simulink model "TV_2017_HIL"  (R2016a)
settings: Solver=ode1  StartTime=0.0  StopTime=600  FixedStep=0.001  RelTol=1e-3
PreLoadFcn:
  | HIL_parameters
values from neighbouring files (symbols this model uses):
  battery_voltage = single(530)    [HIL_parameters.m]    (also in HIL_parameters_2018.m; TV_2017_parameters.m; TV_2017_parameters_VD.m)
  car_params = Simulink_Car_params    [HIL_parameters.m]    (also in HIL_parameters_2018.m; TV_2017_parameters.m; TV_2017_parameters_VD.m)
  i_Diff = 16    [HIL_parameters.m]    (also in HIL_parameters_2018.m; TV_2017_parameters.m)
  Kp = 1    [HIL_parameters.m]    (also in HIL_parameters_2018.m; TV_2017_parameters.m; TV_2017_parameters_VD.m)
  motor_data = struct    [HIL_parameters.m]    (also in HIL_parameters_2018.m; TV_2017_parameters.m)
  settings = Simulink_Settings    [HIL_parameters.m]    (also in HIL_parameters_2018.m; TV_2017_parameters.m; TV_2017_parameters_VD.m)
  SpdC_BCC = 0    [HIL_parameters.m]    (also in HIL_parameters_2018.m; TV_2017_parameters.m; TV_2017_parameters_VD.m)
  Speed_Neg_sat = -21    [HIL_parameters.m]    (also in HIL_parameters_2018.m; TV_2017_parameters.m; TV_2017_parameters_VD.m)
  Speed_Pos_sat = 21    [HIL_parameters.m]    (also in HIL_parameters_2018.m; TV_2017_parameters.m; TV_2017_parameters_VD.m)
  SteeringAngleFL = [-23.80 -22.65 -21.50 -20.34 -19.18 -18.03 -16.86 -15.70 -14.53 -13.35 -12.18 -10.99 -9.80 -8.61 -7.40 -6.19 -4.97 -3.75 -2.51 -1.26 0 1.27 2.56 3.85 5.17 6.50 7.84 9.21 10.59 12.00 13.42 14.88 16.36 17.87 19.41 20.99 22.61 24.26 25.97 27.73 29.54]    [CarSetupAnalysis2018.m]    (also in HIL_parameters_2018.m; TV_2017_parameters.m; TV_2017_parameters_VD.m = [-24.129 -22.950 -21.772 -20.593 -19.413 -18.232 -17.050 -15)
  SteeringAngleFR = [-29.54 -27.73 -25.97 -24.26 -22.61 -20.99 -19.41 -17.87 -16.36 -14.88 -13.42 -12.00 -10.59 -9.21 -7.84 -6.50 -5.17 -3.85 -2.56 -1.27 0 1.26 2.51 3.75 4.97 6.19 7.40 8.61 9.80 10.99 12.18 13.35 14.53 15.70 16.86 18.03 19.18 20.34 21.50 22.65 23.80]    [CarSetupAnalysis2018.m]    (also in HIL_parameters_2018.m; TV_2017_parameters.m; TV_2017_parameters_VD.m = [-29.3050 -27.5340 -25.8140 -24.1410 -22.5110 -20.9180 -19.3)
  SteeringWhAngle = [-105 -99.75 -94.5 -89.25 -84 -78.75 -73.5 -68.25 -63 -57.75 -52.5 -47.25 -42 -36.75 -31.5 -26.25 -21.0 -15.75 -10.5 -5.25 0.0 5.25 10.50 15.75 21.00 26.25 31.50 36.75 42.00 47.25 52.50 57.75  63.00 68.25 73.50 78.75 84.00 89.25 94.50 99.75 105.00]    [TV_2017_parameters_VD.m]
  Tn_n = 0    [HIL_parameters.m]    (also in HIL_parameters_2018.m; TV_2017_parameters.m; TV_2017_parameters_VD.m)
  Use_Joystick = 1    [HIL_parameters.m]    (also in HIL_parameters_2018.m; TV_2017_parameters.m; TV_2017_parameters_VD.m)
undefined symbols (not defined in the file or in its folder): canChannel, TC_Decr_Gas, TC_Derivative, TC_Incr_Gas, TC_On, TC_Relay_Off, TC_Relay_On
libraries: CarMaker4SL x314, canmsglib x48, simulink_extras x48, simulink x41, canlib x39, powerlib_meascontrol x2, sldrtlib x1
(part 2 of 9)

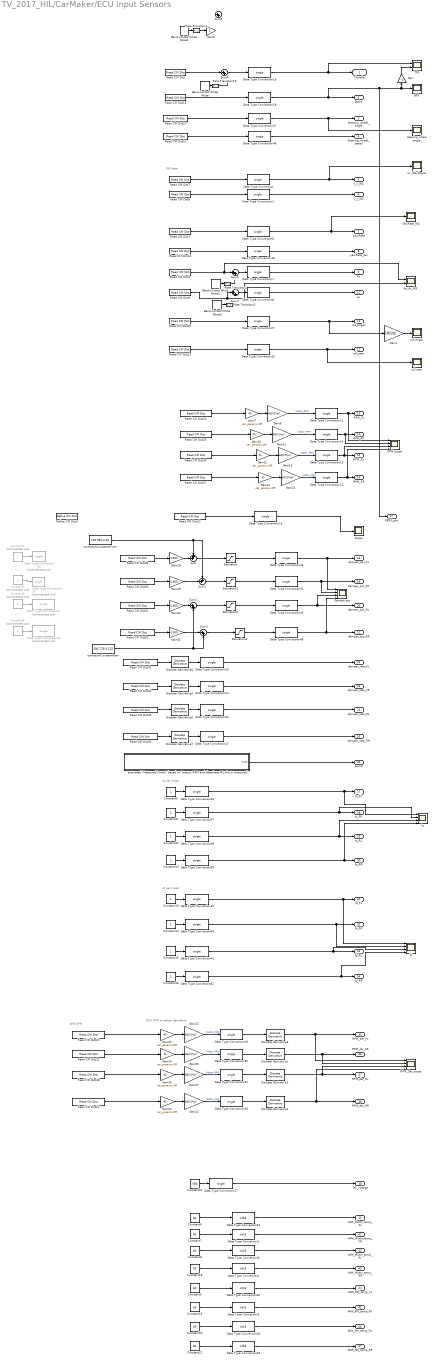
== system TV_2017_HIL/CarMaker/ECU input Sensors  ==
  note: INS data
  note: ECU RPM to radian derivative
  note: AMK RPM
  note: Id per motor
  note: Iq per motor
  Ay_Ax_INS : Scope  NumInputPorts=2
  BPS : Scope
  Band-Limited White Noise : simulink/Sources/Band-Limited White Noise  Cov=[0.00002]  Ts=0.1  seed=[23341]
  Band-Limited White Noise1 : simulink/Sources/Band-Limited White Noise  Cov=[0.00002]  Ts=0.1  seed=[23341]
  Band-Limited White Noise2 : simulink/Sources/Band-Limited White Noise  Cov=[0.01]  Ts=0.1  seed=[23341]
  Band-Limited White Noise3 : simulink/Sources/Band-Limited White Noise  Cov=[0.01]  Ts=0.1  seed=[23341]
  Constant{1..4} (4 alike) : Constant  Commented=on
  Constant{9..16} (8 alike) : Constant
  Constant{5..8,18..20,22} (8 alike) : Constant  Value=60
  Constant21 : Constant  Value=580
  Damper pos : Scope  NumInputPorts=4
  Data Type Conversion{,1,6..19,24..27,32..33,37..52} (38 alike) : DataTypeConversion  OutDataTypeStr=single
  Data Type Conversion{2..5,28..30,54} (8 alike) : DataTypeConversion  OutDataTypeStr=int16
  Data Type Conversion{20..23} (4 alike) : DataTypeConversion  Commented=on  OutDataTypeStr=single
  Define CM Dict3 : CarMaker4SL/Define CM Dict  xname=KERS_pos  xmono=off  xtype=Double  xdvaplace=None  xnstates=0  xfirststate=0  xinitial=0
  Discrete Derivative{1..3,8} (4 alike) : simulink/Discrete/Discrete Derivative  gainval=1.0  ICPrevScaledInput=0.0  InputProcessing=Inherited  OutMin=[]  OutMax=[]  OutDataType=fixdt(1, 16)  OutScaling=2^-10  DoSatur=off
  Discrete Derivative{4..7} (4 alike) : simulink/Discrete/Discrete Derivative  gainval=1.0  ICPrevScaledInput=0.0  OutMin=[]  OutMax=[]  OutDataType=fixdt(1, 16)  OutScaling=2^-10  DoSatur=off
  Gain : Gain  Gain=-1
  Gain1 : Gain  Gain=180/pi
  Gain{7,10,12,14,20,22,24,26} (8 alike) : Gain  Gain=car_params.GR
  Gain{9,11,13,15,21,23,25,27} (8 alike) : Gain  Gain=60/(2*pi)
  Gain2 : Gain
  Gain{28..31} (4 alike) : Gain  Gain=-1000
  Id : Scope  NumInputPorts=4
  Iq : Scope  NumInputPorts=4
  RPM scope : Scope  NumInputPorts=4
  "RPM_Der_scope " : Scope  NumInputPorts=4
  Rate Transition{1..3,19} (4 alike) : RateTransition  OutPortSampleTimeOpt=Inherit  OutPortSampleTime=matlab_params.sensor_sampling_time
  Read CM Dict : CarMaker4SL/Read CM Dict  xname=VC.Gas  xsync=off
  Read CM Dict1 : CarMaker4SL/Read CM Dict  xname=Vhcl.YawRate  xsync=off
  Read CM Dict10 : CarMaker4SL/Read CM Dict  xname=Vhcl.Roll  xsync=off
  Read CM Dict11 : CarMaker4SL/Read CM Dict  xname=Vhcl.RollVel  xsync=off
  Read CM Dict12 : CarMaker4SL/Read CM Dict  xname=KERS_pos  xsync=off
  Read CM Dict13 : CarMaker4SL/Read CM Dict  xname=Vhcl.YawAcc  xsync=off
  Read CM Dict14 : CarMaker4SL/Read CM Dict  xname=Car.WheelSpd_RR  xsync=off
  Read CM Dict15 : CarMaker4SL/Read CM Dict  xname=VC.Brake  xsync=off
  Read CM Dict2 : CarMaker4SL/Read CM Dict  xname=Car.ay  xsync=off
  Read CM Dict20 : CarMaker4SL/Read CM Dict  xname=Vhcl.Steer.Ang  xsync=off
  Read CM Dict21 : CarMaker4SL/Read CM Dict  xname=Vhcl.Steer.Vel  xsync=off
  Read CM Dict22 : CarMaker4SL/Read CM Dict  xname=Car.WheelSpd_FL  xsync=off
  Read CM Dict23 : CarMaker4SL/Read CM Dict  xname=Car.WheelSpd_FR  xsync=off
  Read CM Dict24 : CarMaker4SL/Read CM Dict  xname=Car.WheelSpd_FL  xsync=off
  Read CM Dict25 : CarMaker4SL/Read CM Dict  xname=Car.WheelSpd_FR  xsync=off
  Read CM Dict26 : CarMaker4SL/Read CM Dict  xname=Car.WheelSpd_RL  xsync=off
  Read CM Dict27 : CarMaker4SL/Read CM Dict  xname=Car.WheelSpd_RR  xsync=off
  Read CM Dict28 : CarMaker4SL/Read CM Dict  xname=Car.WheelSpd_RL  xsync=off
  Read CM Dict29 : CarMaker4SL/Read CM Dict  xname=Car.SpringFL.l  xsync=off
  Read CM Dict30 : CarMaker4SL/Read CM Dict  xname=Car.SpringFR.l  xsync=off
  Read CM Dict31 : CarMaker4SL/Read CM Dict  xname=Car.SpringRL.l  xsync=off
  Read CM Dict32 : CarMaker4SL/Read CM Dict  xname=Car.SpringRR.l  xsync=off
  Read CM Dict33 : CarMaker4SL/Read CM Dict  xname=Car.SpringFL.l  xsync=off
  Read CM Dict34 : CarMaker4SL/Read CM Dict  xname=Car.SpringFR.l  xsync=off
  Read CM Dict35 : CarMaker4SL/Read CM Dict  xname=Car.SpringRL.l  xsync=off
  Read CM Dict36 : CarMaker4SL/Read CM Dict  xname=Car.SpringRR.l  xsync=off
  Read CM Dict7 : CarMaker4SL/Read CM Dict  xname=Car.vx  xsync=off
  Read CM Dict8 : CarMaker4SL/Read CM Dict  xname=Car.vy  xsync=off
  Read CM Dict9 : CarMaker4SL/Read CM Dict  xname=Car.ax  xsync=off
  Saturation{,1..3} (4 alike) : Saturate  UpperLimit=200  LowerLimit=0.001
  Scope : Scope
  Sum : Sum  Inputs=++|
  Sum1 : Sum  Inputs=++|
  Sum{2..7} (6 alike) : Sum  Inputs=|++
  TPS : Scope  NumInputPorts=2
  Vx_INS_Scope : Scope
  YawRate_INS : Scope
  correctionConstantRear : Constant  Value=190.725-3.125
  correctionCornstantFront : Constant  Value=190.965-3.63
  "estimated \"Measured Power\" based on Torque, RPM and datasheet IRL this is measured" : Subsystem
  "roll angle " : Scope
  roll rate : Scope
  steering wheel angle : Scope
  "Throttle " : Outport
  "Brake " : Outport  Port=2
  "Steering_wheel_angle " : Outport  Port=3
  Steering_wheel_speed : Outport  Port=4
  V_x_INS : Outport  Port=5
  V_y_INS : Outport  Port=6
  yawRate : Outport  Port=7
  yawRate_der : Outport  Port=8
  ay : Outport  Port=9
  "ax " : Outport  Port=10
  roll_angle : Outport  Port=11
  roll_rate : Outport  Port=12
  RPM_FL : Outport  Port=13
  RPM_FR : Outport  Port=14
  RPM_RL : Outport  Port=15
  RPM_RR : Outport  Port=16
  KERS_pos : Outport  Port=17
  damper_pos_FL : Outport  Port=18
  damper_pos_FR : Outport  Port=19
  damper_pos_RL : Outport  Port=20
  damper_pos_RR : Outport  Port=21
  damper_rate_FL : Outport  Port=22
  damper_rate_FR : Outport  Port=23
  damper_rate_RL : Outport  Port=24
  damper_rate_RR : Outport  Port=25
  power : Outport  Port=26
  Iq_FL : Outport  Port=27
  Iq_FR : Outport  Port=28
  Iq_RL : Outport  Port=29
  Iq_RR : Outport  Port=30
  Id_FL : Outport  Port=31
  Id_FR : Outport  Port=32
  Id_RL : Outport  Port=33
  Id_RR : Outport  Port=34
  RPM_der_FL : Outport  Port=35
  RPM_der_FR : Outport  Port=36
  RPM_der_RL : Outport  Port=37
  RPM_der_RR : Outport  Port=38
  DC_voltage : Outport  Port=39
  AMK_Motor_temp_FL : Outport  Port=40
  AMK_Motor_temp_FR : Outport  Port=41
  AMK_Motor_temp_RL : Outport  Port=42
  AMK_Motor_temp_RR : Outport  Port=43
  AMK_INV_temp_FL : Outport  Port=44
  AMK_INV_temp_FR : Outport  Port=45
  AMK_INV_temp_RL : Outport  Port=46
  AMK_INV_temp_RR : Outport  Port=47
  wires:
  Gain7/1 -> Gain9/1
  Read CM Dict24/1 -> Gain7/1
  Read CM Dict25/1 -> Gain10/1
  Gain10/1 -> Gain11/1
  Gain12/1 -> Gain13/1
  Gain14/1 -> Gain15/1
  Read CM Dict26/1 -> Gain12/1
  Read CM Dict27/1 -> Gain14/1
  Gain9/1 -> Data Type Conversion11/1  "Motor_RPM"
  Gain15/1 -> Data Type Conversion12/1  "Motor_RPM"
  Gain13/1 -> Data Type Conversion13/1  "Motor_RPM"
  Gain11/1 -> Data Type Conversion14/1  "Motor_RPM"
  Data Type Conversion11/1 -> RPM scope/1, RPM_FL/1
  Data Type Conversion14/1 -> RPM scope/2, RPM_FR/1
  Data Type Conversion13/1 -> RPM scope/3, RPM_RL/1
  Data Type Conversion12/1 -> RPM scope/4, RPM_RR/1
  Read CM Dict12/1 -> Data Type Conversion15/1
  Data Type Conversion15/1 -> Scope/1
  Read CM Dict15/1 -> Data Type Conversion18/1
  Data Type Conversion18/1 -> KERS_pos/1, BPS/1, Gain/1, "Brake "/1
  Data Type Conversion19/1 -> TPS/1, "Throttle "/1
  Constant1/1 -> Data Type Conversion21/1
  Constant2/1 -> Data Type Conversion20/1
  Constant3/1 -> Data Type Conversion22/1
  Constant4/1 -> Data Type Conversion23/1
  Data Type Conversion25/1 -> damper_rate_FL/1
  Discrete Derivative4/1 -> Data Type Conversion25/1
  Data Type Conversion24/1 -> damper_rate_FR/1
  Discrete Derivative5/1 -> Data Type Conversion24/1
  Data Type Conversion26/1 -> damper_rate_RL/1
  Discrete Derivative6/1 -> Data Type Conversion26/1
  Data Type Conversion27/1 -> damper_rate_RR/1
  Discrete Derivative7/1 -> Data Type Conversion27/1
  Read CM Dict20/1 -> Data Type Conversion47/1
  Read CM Dict21/1 -> Data Type Conversion48/1
  Data Type Conversion47/1 -> steering wheel angle/1, "Steering_wheel_angle "/1
  Data Type Conversion48/1 -> Steering_wheel_speed/1
  Data Type Conversion17/1 -> DC_voltage/1
  Constant21/1 -> Data Type Conversion17/1
  Read CM Dict30/1 -> Gain29/1
  Read CM Dict31/1 -> Gain30/1
  Read CM Dict32/1 -> Gain31/1
  Read CM Dict29/1 -> Gain28/1
  Data Type Conversion43/1 -> Damper pos/2, damper_pos_FR/1
  Data Type Conversion45/1 -> Damper pos/3, damper_pos_RL/1
  Data Type Conversion44/1 -> Damper pos/1, damper_pos_FL/1
  Data Type Conversion46/1 -> Damper pos/4, damper_pos_RR/1
  Sum/1 -> Saturation/1
  Gain30/1 -> Sum2/1
  Gain31/1 -> Sum3/1
  correctionConstantRear/1 -> Sum3/2, Sum2/2
  Sum1/1 -> Saturation1/1
  Sum2/1 -> Saturation2/1
  Sum3/1 -> Saturation3/1
  Saturation/1 -> Data Type Conversion44/1
  Saturation1/1 -> Data Type Conversion43/1
  Saturation2/1 -> Data Type Conversion45/1
  Saturation3/1 -> Data Type Conversion46/1
  Read CM Dict33/1 -> Discrete Derivative4/1
  Read CM Dict34/1 -> Discrete Derivative5/1
  Read CM Dict35/1 -> Discrete Derivative6/1
  Read CM Dict36/1 -> Discrete Derivative7/1
  Data Type Conversion30/1 -> AMK_INV_temp_FL/1
  Constant5/1 -> Data Type Conversion30/1
  Data Type Conversion54/1 -> AMK_Motor_temp_FL/1
  Constant6/1 -> Data Type Conversion54/1
  Data Type Conversion2/1 -> AMK_Motor_temp_FR/1
  Constant7/1 -> Data Type Conversion2/1
  Data Type Conversion3/1 -> AMK_Motor_temp_RL/1
  Constant8/1 -> Data Type Conversion3/1
  Data Type Conversion4/1 -> AMK_Motor_temp_RR/1
  Constant18/1 -> Data Type Conversion4/1
  Data Type Conversion5/1 -> AMK_INV_temp_FR/1
  Constant19/1 -> Data Type Conversion5/1
  Data Type Conversion28/1 -> AMK_INV_temp_RL/1
  Constant20/1 -> Data Type Conversion28/1
  Data Type Conversion29/1 -> AMK_INV_temp_RR/1
  Constant22/1 -> Data Type Conversion29/1
  Data Type Conversion33/1 -> Iq/1, Iq_FL/1
  Data Type Conversion37/1 -> Iq/2, Iq_FR/1
  Data Type Conversion38/1 -> Iq/3, Iq_RL/1
  Data Type Conversion39/1 -> Iq/4, Iq_RR/1
  Constant11/1 -> Data Type Conversion37/1
  Constant12/1 -> Data Type Conversion38/1
  Constant13/1 -> Data Type Conversion39/1
  Constant9/1 -> Data Type Conversion33/1
  Data Type Conversion32/1 -> Id/1, Id_FL/1
  Data Type Conversion40/1 -> Id/2, Id_FR/1
  Data Type Conversion41/1 -> Id/3, Id_RL/1
  Data Type Conversion42/1 -> Id/4, Id_RR/1
  Constant16/1 -> Data Type Conversion42/1
  Constant14/1 -> Data Type Conversion40/1
  Constant15/1 -> Data Type Conversion41/1
  Constant10/1 -> Data Type Conversion32/1
  Discrete Derivative1/1 -> "RPM_Der_scope "/2, RPM_der_FR/1
  Discrete Derivative2/1 -> "RPM_Der_scope "/3, RPM_der_RL/1
  Discrete Derivative3/1 -> "RPM_Der_scope "/4, RPM_der_RR/1
  Gain21/1 -> Data Type Conversion50/1  "Motor_RPM"
  Gain23/1 -> Data Type Conversion49/1  "Motor_RPM"
  Gain26/1 -> Gain27/1
  Gain25/1 -> Data Type Conversion52/1  "Motor_RPM"
  Data Type Conversion51/1 -> Discrete Derivative2/1
  Gain27/1 -> Data Type Conversion51/1  "Motor_RPM"
  Data Type Conversion52/1 -> Discrete Derivative1/1
  Data Type Conversion50/1 -> Discrete Derivative3/1
  Gain20/1 -> Gain21/1
  Gain24/1 -> Gain25/1
  Gain22/1 -> Gain23/1
  Read CM Dict22/1 -> Gain22/1
  Read CM Dict28/1 -> Gain26/1
  Read CM Dict14/1 -> Gain20/1
  Read CM Dict23/1 -> Gain24/1
  Data Type Conversion10/1 -> roll rate/1, roll_rate/1
  Data Type Conversion9/1 -> Gain1/1, roll_angle/1
  Data Type Conversion/1 -> V_x_INS/1, Vx_INS_Scope/1
  Data Type Conversion1/1 -> V_y_INS/1
  Data Type Conversion6/1 -> yawRate/1, YawRate_INS/1
  Data Type Conversion16/1 -> yawRate_der/1
  Data Type Conversion7/1 -> ay/1
  Data Type Conversion8/1 -> "ax "/1
  Read CM Dict2/1 -> Ay_Ax_INS/1, Sum6/1
  Read CM Dict9/1 -> Sum7/1, Ay_Ax_INS/2
  Read CM Dict13/1 -> Data Type Conversion16/1
  Read CM Dict11/1 -> Data Type Conversion10/1
  Read CM Dict10/1 -> Data Type Conversion9/1
  Read CM Dict8/1 -> Data Type Conversion1/1
  Read CM Dict7/1 -> Data Type Conversion/1
  Read CM Dict1/1 -> Data Type Conversion6/1
  "estimated \"Measured Power\" based on Torque, RPM and datasheet IRL this is measured"/1(Out2) -> power/1
  Gain1/1 -> "roll angle "/1
  Gain28/1 -> Sum/2
  Gain29/1 -> Sum1/2
  correctionCornstantFront/1 -> Sum/1, Sum1/1
  Gain/1 -> TPS/2
  Band-Limited White Noise/1 -> Rate Transition19/1
  Rate Transition19/1 -> ?
  Sum4/1 -> Data Type Conversion19/1
  Read CM Dict/1 -> Sum4/1
  Band-Limited White Noise1/1 -> Rate Transition1/1
  Band-Limited White Noise2/1 -> Rate Transition2/1
  Sum6/1 -> Data Type Conversion7/1
  Band-Limited White Noise3/1 -> Rate Transition3/1
  Sum7/1 -> Data Type Conversion8/1
  Rate Transition1/1 -> Gain2/1
  Rate Transition2/1 -> ?
  Data Type Conversion49/1 -> Discrete Derivative8/1
  Discrete Derivative8/1 -> "RPM_Der_scope "/1, RPM_der_FL/1

== system TV_2017_HIL/CarMaker/Function-Call Subsystem4 ==
  CAN_MSG : Inport
  function : TriggerPort  TriggerType=function-call  VariantControl=Variant
  AMK Inverter Setpoints from ECU : Subsystem  Commented=on
  CAN Unpack1 : canmsglib/CAN Unpack  Commented=on  MsgList=(none)  MsgName=ECU_SET_POINT_FR_ID  MsgIDType=Standard (11-bit identifier)  MsgIdentifier=ECU_SET_POINT_FR_ID  MsgLength=6  SignalInfo=trq_pos$0$16$1$1$1$0$1$0$-Inf$Inf$#trq_neg$16$16$1$1$1$0$1$0$-Inf$Inf$#w_set$32$16$1$1$1$0$1$0$-Inf$Inf$#  NSignals=3  IDPort=off  TimestampPort=on  ErrorPort=off  RemotePort=off  LengthPort=off  StatusPort=off  StartBits=str2num('[int32(0);int32(16);int32(32)]')  SignalSizes=str2num('[int32(16);int32(16);int32(16)]')  ByteOrders=str2num('[int32(1);int32(1);int32(1)]')  DataTypes=str2num('[int32(1);int32(1);int32(1)]')  MultiplexTypes=str2num('[int32(1);int32(1);int32(1)]')  MultiplexValues=str2num('[double(0);double(0);double(0)]')  Factors=str2num('[double(1);double(1);double(1)]')  Offsets=str2num('[double(0);double(0);double(0)]')  Minimums=str2num('[double(-Inf);double(-Inf);double(-Inf)]')  Maximums=str2num('[double(Inf);double(Inf);double(Inf)]')
  CAN Unpack2 : canmsglib/CAN Unpack  Commented=on  MsgList=(none)  MsgName=ECU_SET_POINT_RL_ID  MsgIDType=Standard (11-bit identifier)  MsgIdentifier=ECU_SET_POINT_RL_ID  MsgLength=6  SignalInfo=trq_pos$0$16$1$1$1$0$1$0$-Inf$Inf$#trq_neg$16$16$1$1$1$0$1$0$-Inf$Inf$#w_set$32$16$1$1$1$0$1$0$-Inf$Inf$#  NSignals=3  IDPort=off  TimestampPort=on  ErrorPort=off  RemotePort=off  LengthPort=off  StatusPort=off  StartBits=str2num('[int32(0);int32(16);int32(32)]')  SignalSizes=str2num('[int32(16);int32(16);int32(16)]')  ByteOrders=str2num('[int32(1);int32(1);int32(1)]')  DataTypes=str2num('[int32(1);int32(1);int32(1)]')  MultiplexTypes=str2num('[int32(1);int32(1);int32(1)]')  MultiplexValues=str2num('[double(0);double(0);double(0)]')  Factors=str2num('[double(1);double(1);double(1)]')  Offsets=str2num('[double(0);double(0);double(0)]')  Minimums=str2num('[double(-Inf);double(-Inf);double(-Inf)]')  Maximums=str2num('[double(Inf);double(Inf);double(Inf)]')
  CAN Unpack3 : canmsglib/CAN Unpack  Commented=on  MsgList=(none)  MsgName=ECU_SET_POINT_RR_ID  MsgIDType=Standard (11-bit identifier)  MsgIdentifier=ECU_SET_POINT_RR_ID  MsgLength=6  SignalInfo=trq_pos$0$16$1$1$1$0$1$0$-Inf$Inf$#trq_neg$16$16$1$1$1$0$1$0$-Inf$Inf$#w_set$32$16$1$1$1$0$1$0$-Inf$Inf$#  NSignals=3  IDPort=off  TimestampPort=on  ErrorPort=off  RemotePort=off  LengthPort=off  StatusPort=off  StartBits=str2num('[int32(0);int32(16);int32(32)]')  SignalSizes=str2num('[int32(16);int32(16);int32(16)]')  ByteOrders=str2num('[int32(1);int32(1);int32(1)]')  DataTypes=str2num('[int32(1);int32(1);int32(1)]')  MultiplexTypes=str2num('[int32(1);int32(1);int32(1)]')  MultiplexValues=str2num('[double(0);double(0);double(0)]')  Factors=str2num('[double(1);double(1);double(1)]')  Offsets=str2num('[double(0);double(0);double(0)]')  Minimums=str2num('[double(-Inf);double(-Inf);double(-Inf)]')  Maximums=str2num('[double(Inf);double(Inf);double(Inf)]')
  CAN Unpack4 : canmsglib/CAN Unpack  MsgList=(none)  MsgName=TestTimestamp  MsgIDType=Standard (11-bit identifier)  MsgIdentifier=9  MsgLength=4  SignalInfo=timestamp$0$32$1$2$1$0$1$0$-Inf$Inf$#  NSignals=1  IDPort=off  TimestampPort=on  ErrorPort=off  RemotePort=off  LengthPort=off  StatusPort=off  StartBits=str2num('[int32(0)]')  SignalSizes=str2num('[int32(32)]')  ByteOrders=str2num('[int32(1)]')  DataTypes=str2num('[int32(2)]')  MultiplexTypes=str2num('[int32(1)]')  MultiplexValues=str2num('[double(0)]')  Factors=str2num('[double(1)]')  Offsets=str2num('[double(0)]')  Minimums=str2num('[double(-Inf)]')  Maximums=str2num('[double(Inf)]')
  CAN Unpack5 : canmsglib/CAN Unpack  MsgList=(none)  MsgName=SlipRatios  MsgIDType=Standard (11-bit identifier)  MsgIdentifier=200  MsgLength=8  SignalInfo=SR_FL$0$16$1$1$1$0$1$0$-Inf$Inf$#SR_FR$16$16$1$1$1$0$1$0$-Inf$Inf$#SR_RL$32$16$1$1$1$0$1$0$-Inf$Inf$#SR_RR$48$16$1$1$1$0$1$0$-Inf$Inf$#  NSignals=4  IDPort=off  TimestampPort=on  ErrorPort=off  RemotePort=off  LengthPort=off  StatusPort=off  StartBits=str2num('[int32(0);int32(16);int32(32);int32(48)]')  SignalSizes=str2num('[int32(16);int32(16);int32(16);int32(16)]')  ByteOrders=str2num('[int32(1);int32(1);int32(1);int32(1)]')  DataTypes=str2num('[int32(1);int32(1);int32(1);int32(1)]')  MultiplexTypes=str2num('[int32(1);int32(1);int32(1);int32(1)]')  MultiplexValues=str2num('[double(0);double(0);double(0);double(0)]')  Factors=str2num('[double(1);double(1);double(1);double(1)]')  Offsets=str2num('[double(0);double(0);double(0);double(0)]')  Minimums=str2num('[double(-Inf);double(-Inf);double(-Inf);double(-Inf)]')  Maximums=str2num('[double(Inf);double(Inf);double(Inf);double(Inf)]')
  CAN Unpack6 : canmsglib/CAN Unpack  MsgList=(none)  MsgName=yawRatefeed  MsgIDType=Standard (11-bit identifier)  MsgIdentifier=201  MsgLength=2  SignalInfo=yawRate$0$16$1$1$1$0$1$0$-Inf$Inf$#  NSignals=1  IDPort=off  TimestampPort=on  ErrorPort=off  RemotePort=off  LengthPort=off  StatusPort=off  StartBits=str2num('[int32(0)]')  SignalSizes=str2num('[int32(16)]')  ByteOrders=str2num('[int32(1)]')  DataTypes=str2num('[int32(1)]')  MultiplexTypes=str2num('[int32(1)]')  MultiplexValues=str2num('[double(0)]')  Factors=str2num('[double(1)]')  Offsets=str2num('[double(0)]')  Minimums=str2num('[double(-Inf)]')  Maximums=str2num('[double(Inf)]')
  CAN Unpack7 : canmsglib/CAN Unpack  MsgList=(none)  MsgName=TestTimestamp  MsgIDType=Standard (11-bit identifier)  MsgIdentifier=ECU_FZ_DAMPER_EST_ID  MsgLength=8  SignalInfo=FL_z$0$16$1$2$1$0$1$0$-Inf$Inf$#FR_z$16$16$1$1$1$0$1$0$-Inf$Inf$#RL_z$32$16$1$1$1$0$1$0$-Inf$Inf$#RR_z$48$16$1$1$1$0$1$0$-Inf$Inf$#  NSignals=4  IDPort=off  TimestampPort=on  ErrorPort=off  RemotePort=off  LengthPort=off  StatusPort=off  StartBits=str2num('[int32(0);int32(16);int32(32);int32(48)]')  SignalSizes=str2num('[int32(16);int32(16);int32(16);int32(16)]')  ByteOrders=str2num('[int32(1);int32(1);int32(1);int32(1)]')  DataTypes=str2num('[int32(2);int32(1);int32(1);int32(1)]')  MultiplexTypes=str2num('[int32(1);int32(1);int32(1);int32(1)]')  MultiplexValues=str2num('[double(0);double(0);double(0);double(0)]')  Factors=str2num('[double(1);double(1);double(1);double(1)]')  Offsets=str2num('[double(0);double(0);double(0);double(0)]')  Minimums=str2num('[double(-Inf);double(-Inf);double(-Inf);double(-Inf)]')  Maximums=str2num('[double(Inf);double(Inf);double(Inf);double(Inf)]')
  CAN_SR : Scope
  Fi_z from ECU : Scope  NumInputPorts=4
  From : From  Commented=on
  From1 : From  Commented=on  GotoTag=B
  From2 : From  Commented=on  GotoTag=C
  From3 : From  Commented=on  GotoTag=D
  Gain{,1..3} (4 alike) : Gain  Gain=1/1000
  Gain4 : Gain  Gain=single(0.01)
  Memory : Memory  Commented=on  InheritSampleTime=on
  Mux : Mux  Commented=on
  Mux1 : Mux
  Scope10 : Scope
  Scope11 : Scope  Commented=on
  Scope13 : Scope  Commented=on
  Scope15 : Scope
  Scope7 : Scope  Commented=on
  Scope9 : Scope
  Sum : Sum  Commented=on  Inputs=|-+
  To File : ToFile  Commented=on  Filename=Mat_files_CAN\Can_timestamps.mat  MatrixName=ts  SaveFormat=Timeseries
  To File1 : ToFile  Filename=Mat_files_CAN\testTs.mat  MatrixName=testTs
  To File2 : ToFile  Filename=Mat_files_CAN\Can_SR  MatrixName=sr  SaveFormat=Timeseries
  To File3 : ToFile  Filename=Mat_files_CAN\yawRateRef.mat  MatrixName=rRef  SaveFormat=Timeseries
  yawRateref : Scope
  timestampFL : Outport
  testTs : Outport  Port=2
  wires:
  CAN Unpack3/3 -> ?
  From/1 -> Sum/2, Scope13/1, Memory/1, Mux/1  "t_FL"
  Mux/1 -> To File/1, Scope7/1
  CAN Unpack4/1 -> testTs/1, Scope9/1, To File1/1
  CAN Unpack4/2 -> Scope10/1
  Sum/1 -> Scope11/1, timestampFL/1
  Memory/1 -> Sum/1
  CAN Unpack5/1 -> Gain/1
  Mux1/1 -> CAN_SR/1, To File2/1
  CAN Unpack5/2 -> Gain1/1
  CAN Unpack5/3 -> Gain2/1
  CAN Unpack5/4 -> Gain3/1
  Gain/1 -> Mux1/1
  Gain1/1 -> Mux1/2
  Gain2/1 -> Mux1/3
  Gain3/1 -> Mux1/4
  CAN Unpack6/1 -> Scope15/1, Gain4/1
  Gain4/1 -> yawRateref/1, To File3/1
  From1/1 -> Mux/2
  From2/1 -> Mux/3
  From3/1 -> Mux/4
  CAN_MSG/1 -> AMK Inverter Setpoints from ECU/5(In5), AMK Inverter Setpoints from ECU/6(In6), CAN Unpack7/1, CAN Unpack6/1, CAN Unpack5/1, CAN Unpack4/1, AMK Inverter Setpoints from ECU/2(In2), AMK Inverter Setpoints from ECU/1(In1)
  CAN Unpack7/1 -> Fi_z from ECU/1
  CAN Unpack7/2 -> Fi_z from ECU/2
  CAN Unpack7/3 -> Fi_z from ECU/3
  CAN Unpack7/4 -> Fi_z from ECU/4

== system TV_2017_HIL/CarMaker/IPG Vehicle2 ==
  Sync_In : Inport
  Vhcl.Model.Source : Inport  Port=2
  VhclCtrl.Steering : Inport  Port=3
  Vhcl.Wheel.In : Inport  Port=4
  Vhcl.Misc : Inport  Port=5
  VhclCtrl.Brake : Inport  Port=6
  VhclCtrl.PT : Inport  Port=7
  Brake : Subsystem
  CarAndTrailer : Subsystem
  PowerTrain : Subsystem
  Stop Simulation : Stop
  VehicleSource_BuiltIn : simulink/Logic and Bit Operations/Compare To Constant  relop=~=  const=1  OutDataTypeStr=boolean  ZeroCross=off
  Sync_Out : Outport
  wires:
  VhclCtrl.PT/1 -> PowerTrain/3(VhclCtrl.PT)
  Brake/1(Sync_Out) -> PowerTrain/1(Sync_In)
  CarAndTrailer/1(Sync_Out) -> Brake/1(Sync_In)
  CarAndTrailer/2(Brake.IF.In) -> Brake/2(Brake.IF.In)
  VhclCtrl.Brake/1 -> Brake/3(VhclCtrl.Brake)
  PowerTrain/1(Sync_Out) -> Sync_Out/1
  Vhcl.Misc/1 -> CarAndTrailer/4(Vhcl.Misc)
  Vhcl.Wheel.In/1 -> CarAndTrailer/3(Vhcl.Wheel.In)
  VhclCtrl.Steering/1 -> CarAndTrailer/2(VhclCtrl.Steering)
  Sync_In/1 -> CarAndTrailer/1(Sync_In)
  Vhcl.Model.Source/1 -> VehicleSource_BuiltIn/1
  VehicleSource_BuiltIn/1 -> Stop Simulation/1
  Brake/2(Vhcl.Wheel.PT) -> PowerTrain/2(Vhcl.Wheel.PT)

== system TV_2017_HIL/CarMaker/IPG Vehicle3 ==
  Sync_In : Inport
  Vhcl.Model.Source : Inport  Port=2
  VhclCtrl.Steering : Inport  Port=3
  Vhcl.Wheel.In : Inport  Port=4
  Vhcl.Misc : Inport  Port=5
  VhclCtrl.Brake : Inport  Port=6
  VhclCtrl.PT : Inport  Port=7
  Brake : Subsystem
  CarAndTrailer : Subsystem
  PowerTrain : Subsystem
  Stop Simulation : Stop
  VehicleSource_BuiltIn : simulink/Logic and Bit Operations/Compare To Constant  relop=~=  const=1  OutDataTypeStr=boolean  ZeroCross=off
  Sync_Out : Outport
  wires:
  VhclCtrl.PT/1 -> PowerTrain/3(VhclCtrl.PT)
  Brake/1(Sync_Out) -> PowerTrain/1(Sync_In)
  CarAndTrailer/1(Sync_Out) -> Brake/1(Sync_In)
  CarAndTrailer/2(Brake.IF.In) -> Brake/2(Brake.IF.In)
  VhclCtrl.Brake/1 -> Brake/3(VhclCtrl.Brake)
  PowerTrain/1(Sync_Out) -> Sync_Out/1
  Vhcl.Misc/1 -> CarAndTrailer/4(Vhcl.Misc)
  Vhcl.Wheel.In/1 -> CarAndTrailer/3(Vhcl.Wheel.In)
  VhclCtrl.Steering/1 -> CarAndTrailer/2(VhclCtrl.Steering)
  Sync_In/1 -> CarAndTrailer/1(Sync_In)
  Vhcl.Model.Source/1 -> VehicleSource_BuiltIn/1
  VehicleSource_BuiltIn/1 -> Stop Simulation/1
  Brake/2(Vhcl.Wheel.PT) -> PowerTrain/2(Vhcl.Wheel.PT)

== system TV_2017_HIL/CarMaker/Open GUI ==
  S-Function : S-Function  FunctionName=cm_gui  SFunctionDeploymentMode=off  EnableBusSupport=off
